simulink model "CSE1_Oculus_gesture"  (R2014a)
settings: Solver=ode4  StartTime=0.0  StopTime=inf  FixedStep=0.01  RelTol=1e-3
undefined symbols (not defined in the file): v_max
libraries: marine_gnc x11
(part 1 of 4)
settings Model: Creator=mclab  LastModifiedBy=mclab
settings RTWCC: SystemTargetFile=NIVeriStand_VxWorks.tlc  TemplateMakefile=NIVeriStand_VxWorks.tmf  Description=NI VeriStand VxWorks Real-Time Target for Release 2007b or later  ProcessScript=NIVeriStand_VxWorks_make_rtw_hook
settings STFCustomTargetCC: ConcurrentExecutionCompliant=off  MatFileLogging=on  MATLABClassNameForMDSCustomization=Simulink.SoftwareTarget.TargetSpecificTriggerConfigurationBase  SystemTargetFile=NIVeriStand_VxWorks.tlc

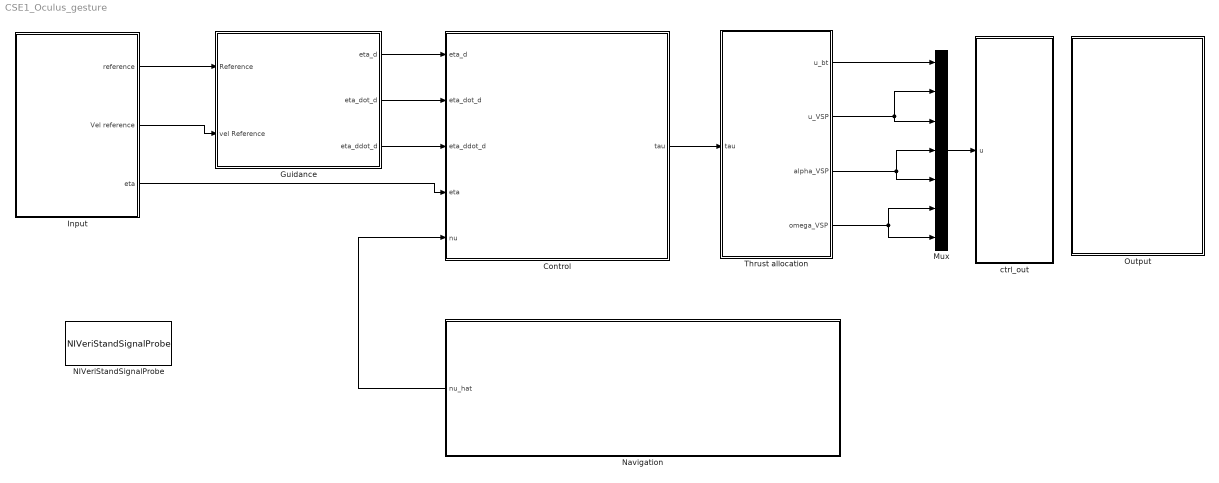
== system CSE1_Oculus_gesture ==
  Control : Subsystem
  Guidance : Subsystem
  Input : Subsystem
  Mux : Mux  Inputs=7
  NIVeriStandSignalProbe : S-Function  FunctionName=NIVeriStandSignalProbe  Parameters=1  EnableBusSupport=off
  "Navigation " : Subsystem
  Output : Subsystem
  Thrust allocation : Subsystem
  ctrl_out : Subsystem
  wires:
  Control/1(tau) -> Thrust allocation/1(tau)
  Input/1(reference) -> Guidance/1("Reference ")
  Guidance/1(eta_d) -> Control/1(eta_d)
  Guidance/3(eta_ddot_d) -> Control/3(eta_ddot_d)
  Guidance/2(eta_dot_d) -> Control/2(eta_dot_d)
  Input/3(eta) -> Control/4(eta)
  Thrust allocation/1(u_bt) -> Mux/1
  Thrust allocation/2(u_VSP) -> Mux/2, Mux/3
  Thrust allocation/3(alpha_VSP) -> Mux/4, Mux/5
  Thrust allocation/4(omega_VSP) -> Mux/6, Mux/7
  "Navigation "/1(nu_hat) -> Control/5(nu)
  Input/2(Vel reference) -> Guidance/2("vel Reference ")
  Mux/1 -> ctrl_out/1(u)

== system CSE1_Oculus_gesture/Control ==
  eta_d : Inport
  eta_dot_d : Inport  Port=2
  eta_ddot_d : Inport  Port=3
  eta : Inport  Port=4
  nu : Inport  Port=5
  DP Controller : Subsystem
  Terminator : Terminator
  tau : Outport
  tag scope: tau=global
  wires:
  eta_d/1 -> DP Controller/1(eta_d)
  eta/1 -> DP Controller/2(eta)
  nu/1 -> DP Controller/3(nu)
  DP Controller/1(tau) -> [tau], tau/1
  eta_ddot_d/1 -> Terminator/1
  eta_dot_d/1 -> DP Controller/4(eta_dot_d)

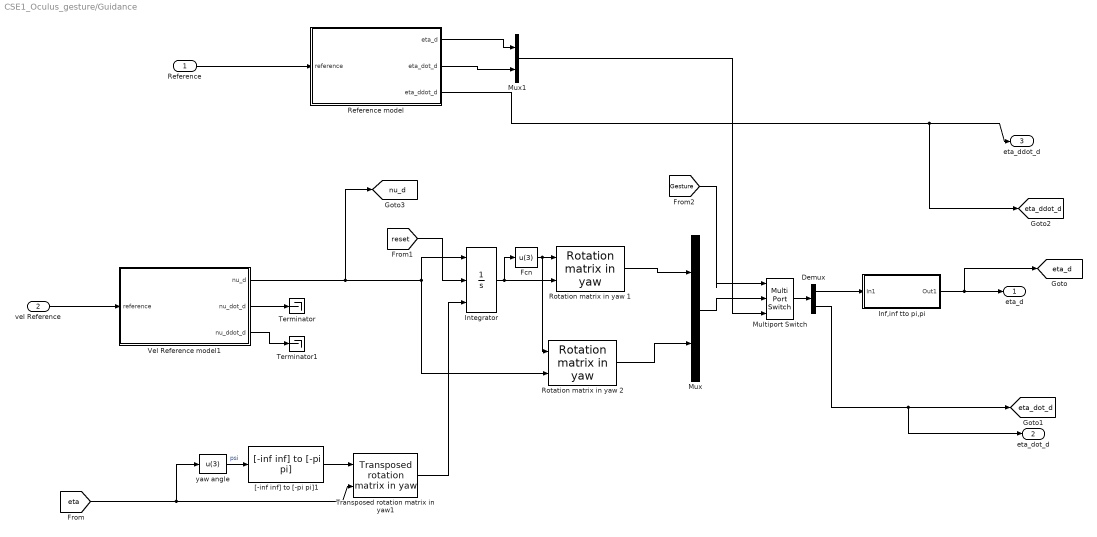
== system CSE1_Oculus_gesture/Guidance ==
  "Reference " : Inport
  "vel Reference " : Inport  Port=2
  Demux : Demux  Outputs=2
  Fcn : Fcn  Expr=u(3)
  Inf,inf tto pi,pi : Subsystem
  Integrator : Integrator  ExternalReset=either  InitialConditionSource=external
  Multiport Switch : MultiPortSwitch  DataPortOrder=Zero-based contiguous  Inputs=2
  Mux : Mux  Inputs=2
  Mux1 : Mux  Inputs=2
  Reference model : Subsystem
  Rotation matrix in yaw 1 : marine_gnc/Models/ Kinematics/Rotation matrix in yaw 
  Rotation matrix in yaw 2 : marine_gnc/Models/ Kinematics/Rotation matrix in yaw 
  Terminator : Terminator
  Terminator1 : Terminator
  Transposed rotation matrix in yaw1 : marine_gnc/Models/ Kinematics/Transposed rotation  matrix in yaw
  Vel Reference model1 : Subsystem
  "[-inf inf] to [-pi pi]1" : marine_gnc/Utilities/Math Operations/[-inf inf] to [-pi pi]
  yaw angle : Fcn  Expr=u(3)
  eta_d : Outport
  eta_dot_d : Outport  Port=2
  eta_ddot_d : Outport  Port=3
  tag scope: eta_d=global, eta_ddot_d=global, eta_dot_d=global, nu_d=global
  wires:
  Demux/1 -> Inf,inf tto pi,pi/1(In1)
  Demux/2 -> eta_dot_d/1, [eta_dot_d]
  Reference model/3(eta_ddot_d) -> [eta_ddot_d], eta_ddot_d/1
  "Reference "/1 -> Reference model/1(reference)
  "vel Reference "/1 -> Vel Reference model1/1(reference)
  Integrator/1 -> Fcn/1, Rotation matrix in yaw 1/2
  Rotation matrix in yaw 1/1 -> Mux/1
  Vel Reference model1/1(nu_d) -> Rotation matrix in yaw 2/2, Integrator/1, [nu_d]
  Fcn/1 -> Rotation matrix in yaw 2/1, Rotation matrix in yaw 1/1
  Rotation matrix in yaw 2/1 -> Mux/2
  Transposed rotation matrix in yaw1/1 -> Integrator/3
  [reset] -> Integrator/2
  "[-inf inf] to [-pi pi]1"/1 -> Transposed rotation matrix in yaw1/1
  yaw angle/1 -> "[-inf inf] to [-pi pi]1"/1  "psi"
  [eta] -> yaw angle/1, Transposed rotation matrix in yaw1/2
  Reference model/2(eta_dot_d) -> Mux1/2
  Reference model/1(eta_d) -> Mux1/1
  Multiport Switch/1 -> Demux/1
  Mux1/1 -> Multiport Switch/3
  Mux/1 -> Multiport Switch/2
  [Gesture] -> Multiport Switch/1
  Vel Reference model1/2(nu_dot_d) -> Terminator/1
  Vel Reference model1/3(nu_ddot_d) -> Terminator1/1
  Inf,inf tto pi,pi/1(Out1) -> [eta_d], eta_d/1

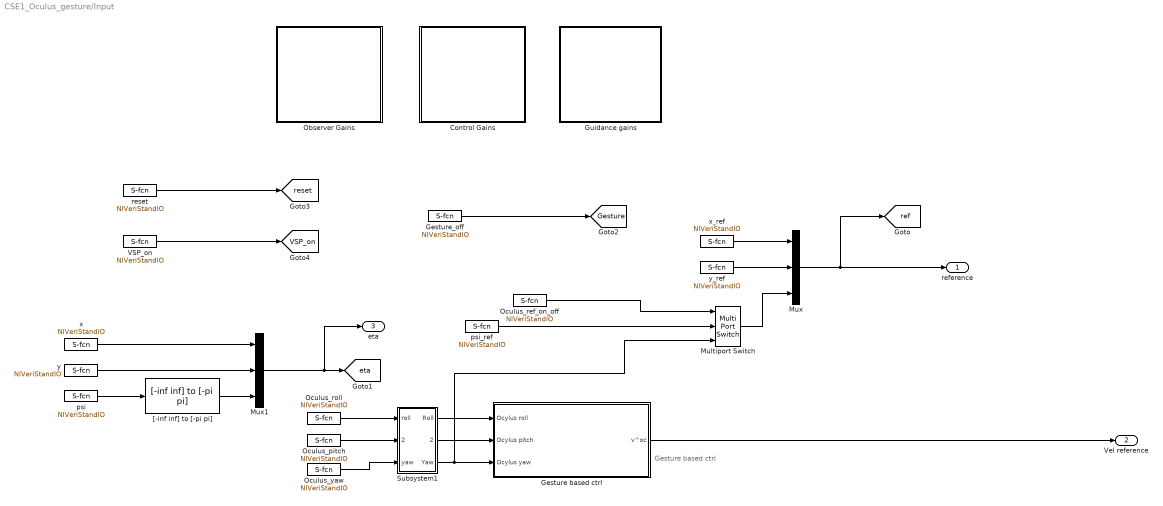
== system CSE1_Oculus_gesture/Input ==
  note: Gesture based ctrl
  Control Gains : Subsystem
  Gesture based ctrl : Subsystem
  Gesture_off : S-Function  Priority=11  FunctionName=NIVeriStandIO  Parameters=width dtype portnum stime stype btype  EnableBusSupport=off  mask(NI VeriStand Inport){portnum=11, width=-1, stime=-1, dtype=auto, stype=auto, btype=1}
      mask prompts: portnum "Port number:"; width "Port dimensions (-1 for dynamically sized):"; stime "Sample time (-1 for inherited):"; dtype "Data type:"; stype "Signal type:"; btype "Block type:"
      mask help: Use this inport on any level of nested subsystems to allow NI VeriStand software to map signals to it.
      mask init:
      | NIVeriStandIO_init;
      settings: CopyFcn=NIVeriStand_MDL_functions('', 'IO_copy');  DeleteFcn=NIVeriStand_MDL_functions('', 'IO_delete');  MoveFcn=set_param(gcb, 'Mask', 'on');
      mask Callback portnum: NIVeriStand_MDL_functions('', 'IO_setportnum');
      mask TypeOptions dtype: auto | double | single | int8 | uint8 | int16 | uint16 | int32 | uint32 | boolean
      mask Callback dtype: NIVeriStand_MDL_functions('', 'IO_booleansignal');
      mask TypeOptions stype: auto | real | complex
      mask Display:
      | patch([-x x], [-y y], [.90980 .81960 .32156]);
      | plot([xrad -x x xrad], [yrad -y y yrad]);
      | fprintf('NI In%d', portnum);
  Guidance gains : Subsystem
  Multiport Switch : MultiPortSwitch  DataPortOrder=Zero-based contiguous  Inputs=2
  Mux : Mux  Inputs=3
  Mux1 : Mux  Inputs=3
  Observer Gains : Subsystem
  Oculus_pitch : S-Function  Priority=12  FunctionName=NIVeriStandIO  Parameters=width dtype portnum stime stype btype  EnableBusSupport=off  mask(NI VeriStand Inport){portnum=12, width=-1, stime=-1, dtype=auto, stype=auto, btype=1}
      mask prompts: portnum "Port number:"; width "Port dimensions (-1 for dynamically sized):"; stime "Sample time (-1 for inherited):"; dtype "Data type:"; stype "Signal type:"; btype "Block type:"
      mask help: Use this inport on any level of nested subsystems to allow NI VeriStand software to map signals to it.
      mask init:
      | NIVeriStandIO_init;
      settings: CopyFcn=NIVeriStand_MDL_functions('', 'IO_copy');  DeleteFcn=NIVeriStand_MDL_functions('', 'IO_delete');  MoveFcn=set_param(gcb, 'Mask', 'on');
      mask Callback portnum: NIVeriStand_MDL_functions('', 'IO_setportnum');
      mask TypeOptions dtype: auto | double | single | int8 | uint8 | int16 | uint16 | int32 | uint32 | boolean
      mask Callback dtype: NIVeriStand_MDL_functions('', 'IO_booleansignal');
      mask TypeOptions stype: auto | real | complex
      mask Display:
      | patch([-x x], [-y y], [.90980 .81960 .32156]);
      | plot([xrad -x x xrad], [yrad -y y yrad]);
      | fprintf('NI In%d', portnum);
  Oculus_ref_on_off : S-Function  Priority=3  FunctionName=NIVeriStandIO  Parameters=width dtype portnum stime stype btype  EnableBusSupport=off  mask(NI VeriStand Inport){portnum=3, width=-1, stime=-1, dtype=auto, stype=auto, btype=1}
      mask prompts: portnum "Port number:"; width "Port dimensions (-1 for dynamically sized):"; stime "Sample time (-1 for inherited):"; dtype "Data type:"; stype "Signal type:"; btype "Block type:"
      mask help: Use this inport on any level of nested subsystems to allow NI VeriStand software to map signals to it.
      mask init:
      | NIVeriStandIO_init;
      settings: CopyFcn=NIVeriStand_MDL_functions('', 'IO_copy');  DeleteFcn=NIVeriStand_MDL_functions('', 'IO_delete');  MoveFcn=set_param(gcb, 'Mask', 'on');
      mask Callback portnum: NIVeriStand_MDL_functions('', 'IO_setportnum');
      mask TypeOptions dtype: auto | double | single | int8 | uint8 | int16 | uint16 | int32 | uint32 | boolean
      mask Callback dtype: NIVeriStand_MDL_functions('', 'IO_booleansignal');
      mask TypeOptions stype: auto | real | complex
      mask Display:
      | patch([-x x], [-y y], [.90980 .81960 .32156]);
      | plot([xrad -x x xrad], [yrad -y y yrad]);
      | fprintf('NI In%d', portnum);
  Oculus_roll : S-Function  Priority=13  FunctionName=NIVeriStandIO  Parameters=width dtype portnum stime stype btype  EnableBusSupport=off  mask(NI VeriStand Inport){portnum=13, width=-1, stime=-1, dtype=auto, stype=auto, btype=1}
      mask prompts: portnum "Port number:"; width "Port dimensions (-1 for dynamically sized):"; stime "Sample time (-1 for inherited):"; dtype "Data type:"; stype "Signal type:"; btype "Block type:"
      mask help: Use this inport on any level of nested subsystems to allow NI VeriStand software to map signals to it.
      mask init:
      | NIVeriStandIO_init;
      settings: CopyFcn=NIVeriStand_MDL_functions('', 'IO_copy');  DeleteFcn=NIVeriStand_MDL_functions('', 'IO_delete');  MoveFcn=set_param(gcb, 'Mask', 'on');
      mask Callback portnum: NIVeriStand_MDL_functions('', 'IO_setportnum');
      mask TypeOptions dtype: auto | double | single | int8 | uint8 | int16 | uint16 | int32 | uint32 | boolean
      mask Callback dtype: NIVeriStand_MDL_functions('', 'IO_booleansignal');
      mask TypeOptions stype: auto | real | complex
      mask Display:
      | patch([-x x], [-y y], [.90980 .81960 .32156]);
      | plot([xrad -x x xrad], [yrad -y y yrad]);
      | fprintf('NI In%d', portnum);
  Oculus_yaw : S-Function  Priority=5  FunctionName=NIVeriStandIO  Parameters=width dtype portnum stime stype btype  EnableBusSupport=off  mask(NI VeriStand Inport){portnum=5, width=-1, stime=-1, dtype=auto, stype=auto, btype=1}
      mask prompts: portnum "Port number:"; width "Port dimensions (-1 for dynamically sized):"; stime "Sample time (-1 for inherited):"; dtype "Data type:"; stype "Signal type:"; btype "Block type:"
      mask help: Use this inport on any level of nested subsystems to allow NI VeriStand software to map signals to it.
      mask init:
      | NIVeriStandIO_init;
      settings: CopyFcn=NIVeriStand_MDL_functions('', 'IO_copy');  DeleteFcn=NIVeriStand_MDL_functions('', 'IO_delete');  MoveFcn=set_param(gcb, 'Mask', 'on');
      mask Callback portnum: NIVeriStand_MDL_functions('', 'IO_setportnum');
      mask TypeOptions dtype: auto | double | single | int8 | uint8 | int16 | uint16 | int32 | uint32 | boolean
      mask Callback dtype: NIVeriStand_MDL_functions('', 'IO_booleansignal');
      mask TypeOptions stype: auto | real | complex
      mask Display:
      | patch([-x x], [-y y], [.90980 .81960 .32156]);
      | plot([xrad -x x xrad], [yrad -y y yrad]);
      | fprintf('NI In%d', portnum);
  Subsystem1 : Subsystem
  VSP_on : S-Function  Priority=2  FunctionName=NIVeriStandIO  Parameters=width dtype portnum stime stype btype  EnableBusSupport=off  mask(NI VeriStand Inport){portnum=2, width=-1, stime=-1, dtype=auto, stype=auto, btype=1}
      mask prompts: portnum "Port number:"; width "Port dimensions (-1 for dynamically sized):"; stime "Sample time (-1 for inherited):"; dtype "Data type:"; stype "Signal type:"; btype "Block type:"
      mask help: Use this inport on any level of nested subsystems to allow NI VeriStand software to map signals to it.
      mask init:
      | NIVeriStandIO_init;
      settings: CopyFcn=NIVeriStand_MDL_functions('', 'IO_copy');  DeleteFcn=NIVeriStand_MDL_functions('', 'IO_delete');  MoveFcn=set_param(gcb, 'Mask', 'on');
      mask Callback portnum: NIVeriStand_MDL_functions('', 'IO_setportnum');
      mask TypeOptions dtype: auto | double | single | int8 | uint8 | int16 | uint16 | int32 | uint32 | boolean
      mask Callback dtype: NIVeriStand_MDL_functions('', 'IO_booleansignal');
      mask TypeOptions stype: auto | real | complex
      mask Display:
      | patch([-x x], [-y y], [.90980 .81960 .32156]);
      | plot([xrad -x x xrad], [yrad -y y yrad]);
      | fprintf('NI In%d', portnum);
  "[-inf inf] to [-pi pi]" : marine_gnc/Utilities/Math Operations/[-inf inf] to [-pi pi]
  psi : S-Function  Priority=10  FunctionName=NIVeriStandIO  Parameters=width dtype portnum stime stype btype  EnableBusSupport=off  mask(NI VeriStand Inport){portnum=10, width=-1, stime=-1, dtype=auto, stype=auto, btype=1}
      mask prompts: portnum "Port number:"; width "Port dimensions (-1 for dynamically sized):"; stime "Sample time (-1 for inherited):"; dtype "Data type:"; stype "Signal type:"; btype "Block type:"
      mask help: Use this inport on any level of nested subsystems to allow NI VeriStand software to map signals to it.
      mask init:
      | NIVeriStandIO_init;
      settings: CopyFcn=NIVeriStand_MDL_functions('', 'IO_copy');  DeleteFcn=NIVeriStand_MDL_functions('', 'IO_delete');  MoveFcn=set_param(gcb, 'Mask', 'on');
      mask Callback portnum: NIVeriStand_MDL_functions('', 'IO_setportnum');
      mask TypeOptions dtype: auto | double | single | int8 | uint8 | int16 | uint16 | int32 | uint32 | boolean
      mask Callback dtype: NIVeriStand_MDL_functions('', 'IO_booleansignal');
      mask TypeOptions stype: auto | real | complex
      mask Display:
      | patch([-x x], [-y y], [.90980 .81960 .32156]);
      | plot([xrad -x x xrad], [yrad -y y yrad]);
      | fprintf('NI In%d', portnum);
  psi_ref : S-Function  Priority=4  FunctionName=NIVeriStandIO  Parameters=width dtype portnum stime stype btype  EnableBusSupport=off  mask(NI VeriStand Inport){portnum=4, width=-1, stime=-1, dtype=auto, stype=auto, btype=1}
      mask prompts: portnum "Port number:"; width "Port dimensions (-1 for dynamically sized):"; stime "Sample time (-1 for inherited):"; dtype "Data type:"; stype "Signal type:"; btype "Block type:"
      mask help: Use this inport on any level of nested subsystems to allow NI VeriStand software to map signals to it.
      mask init:
      | NIVeriStandIO_init;
      settings: CopyFcn=NIVeriStand_MDL_functions('', 'IO_copy');  DeleteFcn=NIVeriStand_MDL_functions('', 'IO_delete');  MoveFcn=set_param(gcb, 'Mask', 'on');
      mask Callback portnum: NIVeriStand_MDL_functions('', 'IO_setportnum');
      mask TypeOptions dtype: auto | double | single | int8 | uint8 | int16 | uint16 | int32 | uint32 | boolean
      mask Callback dtype: NIVeriStand_MDL_functions('', 'IO_booleansignal');
      mask TypeOptions stype: auto | real | complex
      mask Display:
      | patch([-x x], [-y y], [.90980 .81960 .32156]);
      | plot([xrad -x x xrad], [yrad -y y yrad]);
      | fprintf('NI In%d', portnum);
  reset : S-Function  Priority=1  FunctionName=NIVeriStandIO  Parameters=width dtype portnum stime stype btype  EnableBusSupport=off  mask(NI VeriStand Inport){portnum=1, width=-1, stime=-1, dtype=auto, stype=auto, btype=1}
      mask prompts: portnum "Port number:"; width "Port dimensions (-1 for dynamically sized):"; stime "Sample time (-1 for inherited):"; dtype "Data type:"; stype "Signal type:"; btype "Block type:"
      mask help: Use this inport on any level of nested subsystems to allow NI VeriStand software to map signals to it.
      mask init:
      | NIVeriStandIO_init;
      settings: CopyFcn=NIVeriStand_MDL_functions('', 'IO_copy');  DeleteFcn=NIVeriStand_MDL_functions('', 'IO_delete');  MoveFcn=set_param(gcb, 'Mask', 'on');
      mask Callback portnum: NIVeriStand_MDL_functions('', 'IO_setportnum');
      mask TypeOptions dtype: auto | double | single | int8 | uint8 | int16 | uint16 | int32 | uint32 | boolean
      mask Callback dtype: NIVeriStand_MDL_functions('', 'IO_booleansignal');
      mask TypeOptions stype: auto | real | complex
      mask Display:
      | patch([-x x], [-y y], [.90980 .81960 .32156]);
      | plot([xrad -x x xrad], [yrad -y y yrad]);
      | fprintf('NI In%d', portnum);
  x : S-Function  Priority=8  FunctionName=NIVeriStandIO  Parameters=width dtype portnum stime stype btype  EnableBusSupport=off  mask(NI VeriStand Inport){portnum=8, width=-1, stime=-1, dtype=auto, stype=auto, btype=1}
      mask prompts: portnum "Port number:"; width "Port dimensions (-1 for dynamically sized):"; stime "Sample time (-1 for inherited):"; dtype "Data type:"; stype "Signal type:"; btype "Block type:"
      mask help: Use this inport on any level of nested subsystems to allow NI VeriStand software to map signals to it.
      mask init:
      | NIVeriStandIO_init;
      settings: CopyFcn=NIVeriStand_MDL_functions('', 'IO_copy');  DeleteFcn=NIVeriStand_MDL_functions('', 'IO_delete');  MoveFcn=set_param(gcb, 'Mask', 'on');
      mask Callback portnum: NIVeriStand_MDL_functions('', 'IO_setportnum');
      mask TypeOptions dtype: auto | double | single | int8 | uint8 | int16 | uint16 | int32 | uint32 | boolean
      mask Callback dtype: NIVeriStand_MDL_functions('', 'IO_booleansignal');
      mask TypeOptions stype: auto | real | complex
      mask Display:
      | patch([-x x], [-y y], [.90980 .81960 .32156]);
      | plot([xrad -x x xrad], [yrad -y y yrad]);
      | fprintf('NI In%d', portnum);
  x_ref : S-Function  Priority=6  FunctionName=NIVeriStandIO  Parameters=width dtype portnum stime stype btype  EnableBusSupport=off  mask(NI VeriStand Inport){portnum=6, width=-1, stime=-1, dtype=auto, stype=auto, btype=1}
      mask prompts: portnum "Port number:"; width "Port dimensions (-1 for dynamically sized):"; stime "Sample time (-1 for inherited):"; dtype "Data type:"; stype "Signal type:"; btype "Block type:"
      mask help: Use this inport on any level of nested subsystems to allow NI VeriStand software to map signals to it.
      mask init:
      | NIVeriStandIO_init;
      settings: CopyFcn=NIVeriStand_MDL_functions('', 'IO_copy');  DeleteFcn=NIVeriStand_MDL_functions('', 'IO_delete');  MoveFcn=set_param(gcb, 'Mask', 'on');
      mask Callback portnum: NIVeriStand_MDL_functions('', 'IO_setportnum');
      mask TypeOptions dtype: auto | double | single | int8 | uint8 | int16 | uint16 | int32 | uint32 | boolean
      mask Callback dtype: NIVeriStand_MDL_functions('', 'IO_booleansignal');
      mask TypeOptions stype: auto | real | complex
      mask Display:
      | patch([-x x], [-y y], [.90980 .81960 .32156]);
      | plot([xrad -x x xrad], [yrad -y y yrad]);
      | fprintf('NI In%d', portnum);
  y : S-Function  Priority=9  FunctionName=NIVeriStandIO  Parameters=width dtype portnum stime stype btype  EnableBusSupport=off  mask(NI VeriStand Inport){portnum=9, width=-1, stime=-1, dtype=auto, stype=auto, btype=1}
      mask prompts: portnum "Port number:"; width "Port dimensions (-1 for dynamically sized):"; stime "Sample time (-1 for inherited):"; dtype "Data type:"; stype "Signal type:"; btype "Block type:"
      mask help: Use this inport on any level of nested subsystems to allow NI VeriStand software to map signals to it.
      mask init:
      | NIVeriStandIO_init;
      settings: CopyFcn=NIVeriStand_MDL_functions('', 'IO_copy');  DeleteFcn=NIVeriStand_MDL_functions('', 'IO_delete');  MoveFcn=set_param(gcb, 'Mask', 'on');
      mask Callback portnum: NIVeriStand_MDL_functions('', 'IO_setportnum');
      mask TypeOptions dtype: auto | double | single | int8 | uint8 | int16 | uint16 | int32 | uint32 | boolean
      mask Callback dtype: NIVeriStand_MDL_functions('', 'IO_booleansignal');
      mask TypeOptions stype: auto | real | complex
      mask Display:
      | patch([-x x], [-y y], [.90980 .81960 .32156]);
      | plot([xrad -x x xrad], [yrad -y y yrad]);
      | fprintf('NI In%d', portnum);
  y_ref : S-Function  Priority=7  FunctionName=NIVeriStandIO  Parameters=width dtype portnum stime stype btype  EnableBusSupport=off  mask(NI VeriStand Inport){portnum=7, width=-1, stime=-1, dtype=auto, stype=auto, btype=1}
      mask prompts: portnum "Port number:"; width "Port dimensions (-1 for dynamically sized):"; stime "Sample time (-1 for inherited):"; dtype "Data type:"; stype "Signal type:"; btype "Block type:"
      mask help: Use this inport on any level of nested subsystems to allow NI VeriStand software to map signals to it.
      mask init:
      | NIVeriStandIO_init;
      settings: CopyFcn=NIVeriStand_MDL_functions('', 'IO_copy');  DeleteFcn=NIVeriStand_MDL_functions('', 'IO_delete');  MoveFcn=set_param(gcb, 'Mask', 'on');
      mask Callback portnum: NIVeriStand_MDL_functions('', 'IO_setportnum');
      mask TypeOptions dtype: auto | double | single | int8 | uint8 | int16 | uint16 | int32 | uint32 | boolean
      mask Callback dtype: NIVeriStand_MDL_functions('', 'IO_booleansignal');
      mask TypeOptions stype: auto | real | complex
      mask Display:
      | patch([-x x], [-y y], [.90980 .81960 .32156]);
      | plot([xrad -x x xrad], [yrad -y y yrad]);
      | fprintf('NI In%d', portnum);
  reference : Outport
  Vel reference : Outport  Port=2
  eta : Outport  Port=3
  tag scope: Gesture=global, VSP_on=global, eta=global, ref=global, reset=global
  wires:
  Mux/1 -> [ref], reference/1
  reset/1 -> [reset]
  VSP_on/1 -> [VSP_on]
  x_ref/1 -> Mux/1
  y_ref/1 -> Mux/2
  psi_ref/1 -> Multiport Switch/2
  psi/1 -> "[-inf inf] to [-pi pi]"/1
  Mux1/1 -> eta/1, [eta]
  Multiport Switch/1 -> Mux/3
  Oculus_ref_on_off/1 -> Multiport Switch/1
  y/1 -> Mux1/2
  x/1 -> Mux1/1
  Gesture based ctrl/1("v^oc ") -> Vel reference/1
  Gesture_off/1 -> [Gesture]
  "[-inf inf] to [-pi pi]"/1 -> Mux1/3
  Subsystem1/3(Yaw) -> Multiport Switch/3, Gesture based ctrl/3(Ocylus yaw)
  Oculus_roll/1 -> Subsystem1/1(roll)
  Oculus_pitch/1 -> Subsystem1/2(pitch)
  Oculus_yaw/1 -> Subsystem1/3(yaw)
  Subsystem1/1(Roll) -> Gesture based ctrl/1(Ocylus roll)
  Subsystem1/2(Pitch) -> Gesture based ctrl/2(Ocylus pitch)

== system CSE1_Oculus_gesture/Navigation  ==
  Derivative filter : Subsystem
  nu_hat : Outport
  tag scope: nu_hat=global
  wires:
  [eta] -> Derivative filter/1(eta)
  Derivative filter/1(nu_hat) -> nu_hat/1, [nu_hat]

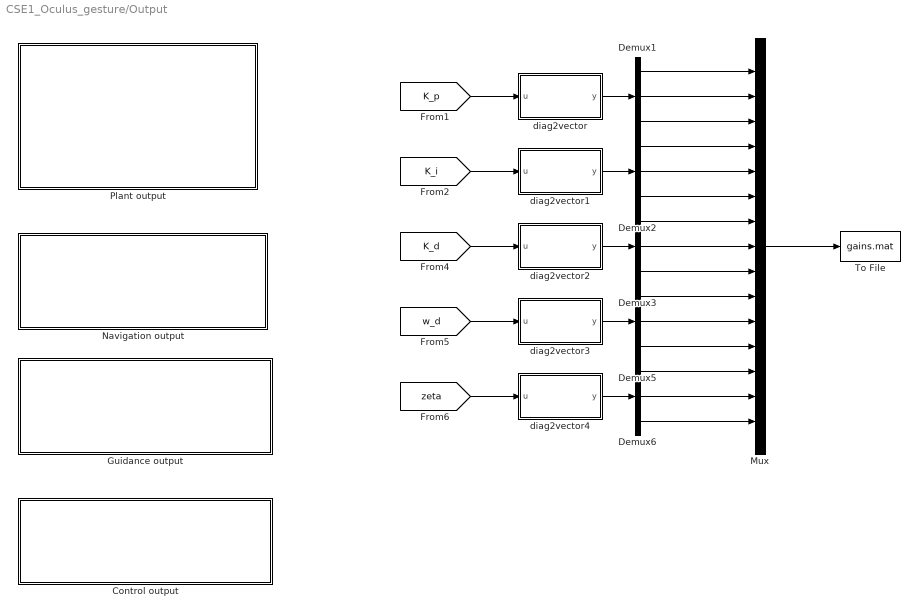
== system CSE1_Oculus_gesture/Output ==
  Control output : Subsystem
  Demux{1..3,5..6} (5 alike) : Demux  Outputs=3
  Guidance output : Subsystem
  Mux : Mux  Inputs=15
  Navigation output : Subsystem
  Plant output : Subsystem
  To File : ToFile  Filename=gains.mat
  diag2vector : MATLAB Function  TreatAsAtomicUnit=on
  diag2vector1 : MATLAB Function  TreatAsAtomicUnit=on
  diag2vector2 : MATLAB Function  TreatAsAtomicUnit=on
  diag2vector3 : MATLAB Function  TreatAsAtomicUnit=on
  diag2vector4 : MATLAB Function  TreatAsAtomicUnit=on
  wires:
  Mux/1 -> To File/1
  [K_p] -> diag2vector/1(u)
  diag2vector/1(y) -> Demux1/1
  Demux1/1 -> Mux/1
  Demux1/2 -> Mux/2
  Demux1/3 -> Mux/3
  [K_i] -> diag2vector1/1(u)
  diag2vector1/1(y) -> Demux2/1
  Demux2/1 -> Mux/4
  Demux2/2 -> Mux/5
  Demux2/3 -> Mux/6
  [K_d] -> diag2vector2/1(u)
  diag2vector2/1(y) -> Demux3/1
  Demux3/1 -> Mux/7
  Demux3/2 -> Mux/8
  Demux3/3 -> Mux/9
  [w_d] -> diag2vector3/1(u)
  diag2vector3/1(y) -> Demux5/1
  Demux5/1 -> Mux/10
  Demux5/2 -> Mux/11
  Demux5/3 -> Mux/12
  [zeta] -> diag2vector4/1(u)
  diag2vector4/1(y) -> Demux6/1
  Demux6/1 -> Mux/13
  Demux6/2 -> Mux/14
  Demux6/3 -> Mux/15

== system CSE1_Oculus_gesture/Thrust allocation ==
  tau : Inport
  Demux : Demux  Outputs=3
  Mux1 : Mux  Inputs=3
  Thrust allocation : MATLAB Function  TreatAsAtomicUnit=on
  u_bt : Outport
  u_VSP : Outport  Port=2
  alpha_VSP : Outport  Port=3
  omega_VSP : Outport  Port=4
  tag scope: thrust=global
  wires:
  [VSP_on] -> Thrust allocation/4(VSP_on)
  Demux/1 -> Thrust allocation/1(X)
  Demux/3 -> Thrust allocation/3(N)
  Thrust allocation/4(omega_VSP) -> omega_VSP/1
  Demux/2 -> Thrust allocation/2(Y)
  tau/1 -> Demux/1
  Thrust allocation/1(u_BT) -> u_bt/1, Mux1/1
  Thrust allocation/2(u_VSP) -> u_VSP/1, Mux1/2
  Thrust allocation/3(alpha_VSP) -> alpha_VSP/1, Mux1/3
  Mux1/1 -> [thrust]

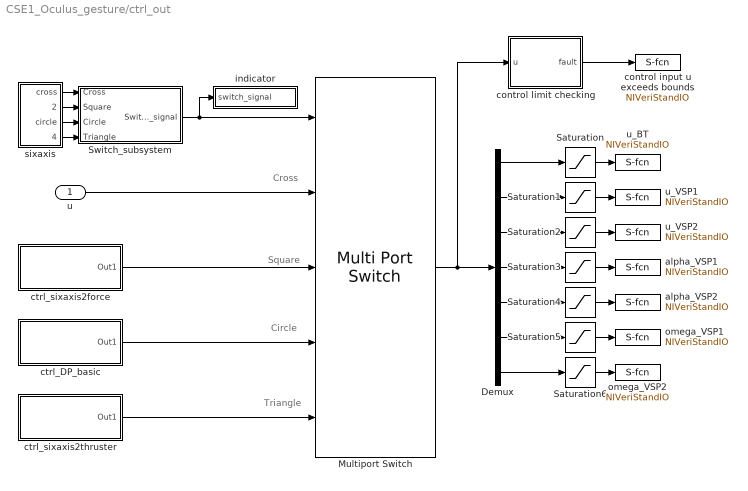
== system CSE1_Oculus_gesture/ctrl_out ==
  note: Cross
  note: Square
  note: Circle
  note: Triangle
  u : Inport
  Demux : Demux  Outputs=7
  Multiport Switch : MultiPortSwitch  Inputs=4
  Saturation : Saturate  UpperLimit=1  LowerLimit=-1
  Saturation1 : Saturate  UpperLimit=1  LowerLimit=0
  Saturation2 : Saturate  UpperLimit=1  LowerLimit=0
  Saturation3 : Saturate  UpperLimit=pi  LowerLimit=-pi
  Saturation4 : Saturate  UpperLimit=pi  LowerLimit=-pi
  Saturation5 : Saturate  UpperLimit=1  LowerLimit=-1
  Saturation6 : Saturate  UpperLimit=1  LowerLimit=-1
  Switch_subsystem : Subsystem
  alpha_VSP1 : S-Function  Priority=5  FunctionName=NIVeriStandIO  Parameters=width dtype portnum stime stype btype  EnableBusSupport=off  mask(NI VeriStand Outport){portnum=5, width=-1, stime=-1, dtype=auto, stype=auto, btype=0}
      mask prompts: portnum "Port number:"; width "Port dimensions (-1 for dynamically sized):"; stime "Sample time (-1 for inherited):"; dtype "Data type:"; stype "Signal type:"; btype "Block type:"
      mask help: Use this outport on any level of nested subsystems to allow NI VeriStand software to map signals to it.
      mask init:
      | NIVeriStandIO_init;
      settings: CopyFcn=NIVeriStand_MDL_functions('', 'IO_copy');  DeleteFcn=NIVeriStand_MDL_functions('', 'IO_delete');  MoveFcn=set_param(gcb, 'Mask', 'on');
      mask Callback portnum: NIVeriStand_MDL_functions('', 'IO_setportnum');
      mask TypeOptions dtype: auto | double | single | int8 | uint8 | int16 | uint16 | int32 | uint32 | boolean
      mask Callback dtype: NIVeriStand_MDL_functions('', 'IO_booleansignal');
      mask TypeOptions stype: auto | real | complex
      mask Display:
      | patch([-x x], [-y y], [.90980 .81960 .32156]);
      | plot([xrad -x x xrad], [yrad -y y yrad]);
      | fprintf('NI Out%d', portnum);
  alpha_VSP2 : S-Function  Priority=1  FunctionName=NIVeriStandIO  Parameters=width dtype portnum stime stype btype  EnableBusSupport=off  mask(NI VeriStand Outport){portnum=1, width=-1, stime=-1, dtype=auto, stype=auto, btype=0}
      mask prompts: portnum "Port number:"; width "Port dimensions (-1 for dynamically sized):"; stime "Sample time (-1 for inherited):"; dtype "Data type:"; stype "Signal type:"; btype "Block type:"
      mask help: Use this outport on any level of nested subsystems to allow NI VeriStand software to map signals to it.
      mask init:
      | NIVeriStandIO_init;
      settings: CopyFcn=NIVeriStand_MDL_functions('', 'IO_copy');  DeleteFcn=NIVeriStand_MDL_functions('', 'IO_delete');  MoveFcn=set_param(gcb, 'Mask', 'on');
      mask Callback portnum: NIVeriStand_MDL_functions('', 'IO_setportnum');
      mask TypeOptions dtype: auto | double | single | int8 | uint8 | int16 | uint16 | int32 | uint32 | boolean
      mask Callback dtype: NIVeriStand_MDL_functions('', 'IO_booleansignal');
      mask TypeOptions stype: auto | real | complex
      mask Display:
      | patch([-x x], [-y y], [.90980 .81960 .32156]);
      | plot([xrad -x x xrad], [yrad -y y yrad]);
      | fprintf('NI Out%d', portnum);
  control input u exceeds bounds : S-Function  Priority=8  FunctionName=NIVeriStandIO  Parameters=width dtype portnum stime stype btype  EnableBusSupport=off  mask(NI VeriStand Outport){portnum=8, width=-1, stime=-1, dtype=auto, stype=auto, btype=0}
      mask prompts: portnum "Port number:"; width "Port dimensions (-1 for dynamically sized):"; stime "Sample time (-1 for inherited):"; dtype "Data type:"; stype "Signal type:"; btype "Block type:"
      mask help: Use this outport on any level of nested subsystems to allow NI VeriStand software to map signals to it.
      mask init:
      | NIVeriStandIO_init;
      settings: CopyFcn=NIVeriStand_MDL_functions('', 'IO_copy');  DeleteFcn=NIVeriStand_MDL_functions('', 'IO_delete');  MoveFcn=set_param(gcb, 'Mask', 'on');
      mask Callback portnum: NIVeriStand_MDL_functions('', 'IO_setportnum');
      mask TypeOptions dtype: auto | double | single | int8 | uint8 | int16 | uint16 | int32 | uint32 | boolean
      mask Callback dtype: NIVeriStand_MDL_functions('', 'IO_booleansignal');
      mask TypeOptions stype: auto | real | complex
      mask Display:
      | patch([-x x], [-y y], [.90980 .81960 .32156]);
      | plot([xrad -x x xrad], [yrad -y y yrad]);
      | fprintf('NI Out%d', portnum);
  control limit checking : MATLAB Function  TreatAsAtomicUnit=on
  ctrl_DP_basic : Subsystem
  ctrl_sixaxis2force : Subsystem
  ctrl_sixaxis2thruster : Subsystem
  indicator : Subsystem
  omega_VSP1 : S-Function  Priority=6  FunctionName=NIVeriStandIO  Parameters=width dtype portnum stime stype btype  EnableBusSupport=off  mask(NI VeriStand Outport){portnum=6, width=-1, stime=-1, dtype=auto, stype=auto, btype=0}
      mask prompts: portnum "Port number:"; width "Port dimensions (-1 for dynamically sized):"; stime "Sample time (-1 for inherited):"; dtype "Data type:"; stype "Signal type:"; btype "Block type:"
      mask help: Use this outport on any level of nested subsystems to allow NI VeriStand software to map signals to it.
      mask init:
      | NIVeriStandIO_init;
      settings: CopyFcn=NIVeriStand_MDL_functions('', 'IO_copy');  DeleteFcn=NIVeriStand_MDL_functions('', 'IO_delete');  MoveFcn=set_param(gcb, 'Mask', 'on');
      mask Callback portnum: NIVeriStand_MDL_functions('', 'IO_setportnum');
      mask TypeOptions dtype: auto | double | single | int8 | uint8 | int16 | uint16 | int32 | uint32 | boolean
      mask Callback dtype: NIVeriStand_MDL_functions('', 'IO_booleansignal');
      mask TypeOptions stype: auto | real | complex
      mask Display:
      | patch([-x x], [-y y], [.90980 .81960 .32156]);
      | plot([xrad -x x xrad], [yrad -y y yrad]);
      | fprintf('NI Out%d', portnum);
  omega_VSP2 : S-Function  Priority=7  FunctionName=NIVeriStandIO  Parameters=width dtype portnum stime stype btype  EnableBusSupport=off  mask(NI VeriStand Outport){portnum=7, width=-1, stime=-1, dtype=auto, stype=auto, btype=0}
      mask prompts: portnum "Port number:"; width "Port dimensions (-1 for dynamically sized):"; stime "Sample time (-1 for inherited):"; dtype "Data type:"; stype "Signal type:"; btype "Block type:"
      mask help: Use this outport on any level of nested subsystems to allow NI VeriStand software to map signals to it.
      mask init:
      | NIVeriStandIO_init;
      settings: CopyFcn=NIVeriStand_MDL_functions('', 'IO_copy');  DeleteFcn=NIVeriStand_MDL_functions('', 'IO_delete');  MoveFcn=set_param(gcb, 'Mask', 'on');
      mask Callback portnum: NIVeriStand_MDL_functions('', 'IO_setportnum');
      mask TypeOptions dtype: auto | double | single | int8 | uint8 | int16 | uint16 | int32 | uint32 | boolean
      mask Callback dtype: NIVeriStand_MDL_functions('', 'IO_booleansignal');
      mask TypeOptions stype: auto | real | complex
      mask Display:
      | patch([-x x], [-y y], [.90980 .81960 .32156]);
      | plot([xrad -x x xrad], [yrad -y y yrad]);
      | fprintf('NI Out%d', portnum);
  sixaxis : Subsystem
  u_BT : S-Function  Priority=2  FunctionName=NIVeriStandIO  Parameters=width dtype portnum stime stype btype  EnableBusSupport=off  mask(NI VeriStand Outport){portnum=2, width=-1, stime=-1, dtype=auto, stype=auto, btype=0}
      mask prompts: portnum "Port number:"; width "Port dimensions (-1 for dynamically sized):"; stime "Sample time (-1 for inherited):"; dtype "Data type:"; stype "Signal type:"; btype "Block type:"
      mask help: Use this outport on any level of nested subsystems to allow NI VeriStand software to map signals to it.
      mask init:
      | NIVeriStandIO_init;
      settings: CopyFcn=NIVeriStand_MDL_functions('', 'IO_copy');  DeleteFcn=NIVeriStand_MDL_functions('', 'IO_delete');  MoveFcn=set_param(gcb, 'Mask', 'on');
      mask Callback portnum: NIVeriStand_MDL_functions('', 'IO_setportnum');
      mask TypeOptions dtype: auto | double | single | int8 | uint8 | int16 | uint16 | int32 | uint32 | boolean
      mask Callback dtype: NIVeriStand_MDL_functions('', 'IO_booleansignal');
      mask TypeOptions stype: auto | real | complex
      mask Display:
      | patch([-x x], [-y y], [.90980 .81960 .32156]);
      | plot([xrad -x x xrad], [yrad -y y yrad]);
      | fprintf('NI Out%d', portnum);
  u_VSP1 : S-Function  Priority=3  FunctionName=NIVeriStandIO  Parameters=width dtype portnum stime stype btype  EnableBusSupport=off  mask(NI VeriStand Outport){portnum=3, width=-1, stime=-1, dtype=auto, stype=auto, btype=0}
      mask prompts: portnum "Port number:"; width "Port dimensions (-1 for dynamically sized):"; stime "Sample time (-1 for inherited):"; dtype "Data type:"; stype "Signal type:"; btype "Block type:"
      mask help: Use this outport on any level of nested subsystems to allow NI VeriStand software to map signals to it.
      mask init:
      | NIVeriStandIO_init;
      settings: CopyFcn=NIVeriStand_MDL_functions('', 'IO_copy');  DeleteFcn=NIVeriStand_MDL_functions('', 'IO_delete');  MoveFcn=set_param(gcb, 'Mask', 'on');
      mask Callback portnum: NIVeriStand_MDL_functions('', 'IO_setportnum');
      mask TypeOptions dtype: auto | double | single | int8 | uint8 | int16 | uint16 | int32 | uint32 | boolean
      mask Callback dtype: NIVeriStand_MDL_functions('', 'IO_booleansignal');
      mask TypeOptions stype: auto | real | complex
      mask Display:
      | patch([-x x], [-y y], [.90980 .81960 .32156]);
      | plot([xrad -x x xrad], [yrad -y y yrad]);
      | fprintf('NI Out%d', portnum);
  u_VSP2 : S-Function  Priority=4  FunctionName=NIVeriStandIO  Parameters=width dtype portnum stime stype btype  EnableBusSupport=off  mask(NI VeriStand Outport){portnum=4, width=-1, stime=-1, dtype=auto, stype=auto, btype=0}
      mask prompts: portnum "Port number:"; width "Port dimensions (-1 for dynamically sized):"; stime "Sample time (-1 for inherited):"; dtype "Data type:"; stype "Signal type:"; btype "Block type:"
      mask help: Use this outport on any level of nested subsystems to allow NI VeriStand software to map signals to it.
      mask init:
      | NIVeriStandIO_init;
      settings: CopyFcn=NIVeriStand_MDL_functions('', 'IO_copy');  DeleteFcn=NIVeriStand_MDL_functions('', 'IO_delete');  MoveFcn=set_param(gcb, 'Mask', 'on');
      mask Callback portnum: NIVeriStand_MDL_functions('', 'IO_setportnum');
      mask TypeOptions dtype: auto | double | single | int8 | uint8 | int16 | uint16 | int32 | uint32 | boolean
      mask Callback dtype: NIVeriStand_MDL_functions('', 'IO_booleansignal');
      mask TypeOptions stype: auto | real | complex
      mask Display:
      | patch([-x x], [-y y], [.90980 .81960 .32156]);
      | plot([xrad -x x xrad], [yrad -y y yrad]);
      | fprintf('NI Out%d', portnum);
  wires:
  Multiport Switch/1 -> control limit checking/1(u), Demux/1
  Demux/1 -> Saturation/1
  Demux/2 -> Saturation1/1
  Demux/3 -> Saturation2/1
  Demux/4 -> Saturation3/1
  Demux/5 -> Saturation4/1
  Demux/6 -> Saturation5/1
  Demux/7 -> Saturation6/1
  Switch_subsystem/1(Switch_signal) -> indicator/1(switch_signal), Multiport Switch/1
  ctrl_sixaxis2thruster/1(Out1) -> Multiport Switch/5
  ctrl_DP_basic/1(Out1) -> Multiport Switch/4
  ctrl_sixaxis2force/1(Out1) -> Multiport Switch/3
  sixaxis/1(cross) -> Switch_subsystem/1(Cross)
  sixaxis/2(square) -> Switch_subsystem/2(Square)
  sixaxis/3(circle) -> Switch_subsystem/3(Circle)
  sixaxis/4(triangle) -> Switch_subsystem/4(Triangle)
  Saturation/1 -> u_BT/1
  Saturation1/1 -> u_VSP1/1
  Saturation2/1 -> u_VSP2/1
  Saturation3/1 -> alpha_VSP1/1
  Saturation4/1 -> alpha_VSP2/1
  Saturation5/1 -> omega_VSP1/1
  Saturation6/1 -> omega_VSP2/1
  control limit checking/1(fault) -> control input u exceeds bounds/1
  u/1 -> Multiport Switch/2

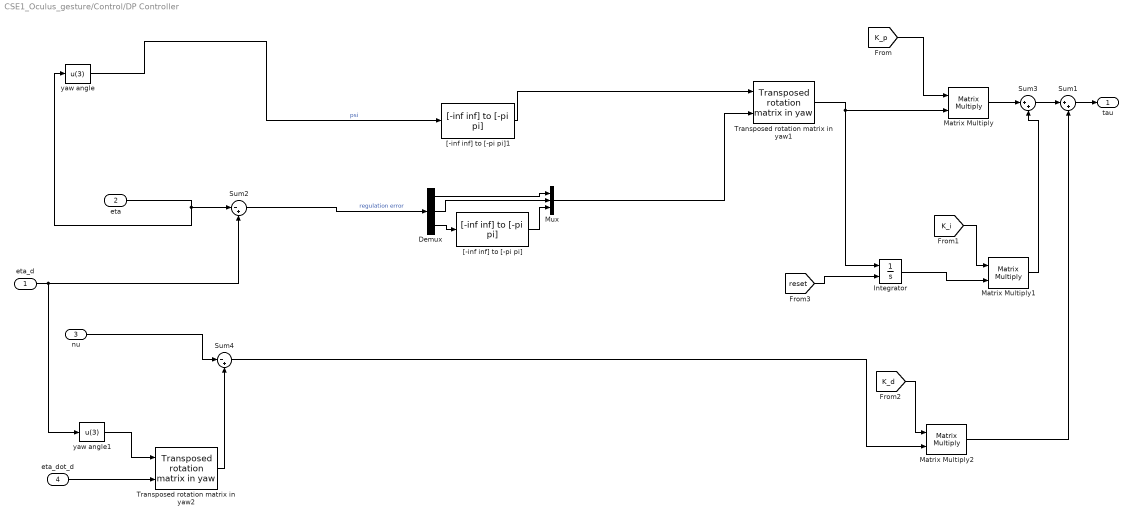
== system CSE1_Oculus_gesture/Control/DP Controller ==
  eta_d : Inport
  eta : Inport  Port=2
  nu : Inport  Port=3
  eta_dot_d : Inport  Port=4
  Demux : Demux  Outputs=3
  Integrator : Integrator  ExternalReset=either
  Matrix Multiply : Product  Multiplication=Matrix(*)
  Matrix Multiply1 : Product  Multiplication=Matrix(*)
  Matrix Multiply2 : Product  Multiplication=Matrix(*)
  Mux : Mux  Inputs=3
  Sum1 : Sum  Inputs=|++  SaturateOnIntegerOverflow=on  InputSameDT=on  OutDataTypeStr=Inherit: Same as first input
  Sum2 : Sum  Inputs=|-+  SaturateOnIntegerOverflow=on  InputSameDT=on  OutDataTypeStr=Inherit: Same as first input
  Sum3 : Sum  Inputs=|++  SaturateOnIntegerOverflow=on  InputSameDT=on  OutDataTypeStr=Inherit: Same as first input
  Sum4 : Sum  Inputs=|-+  SaturateOnIntegerOverflow=on  InputSameDT=on  OutDataTypeStr=Inherit: Same as first input
  Transposed rotation matrix in yaw1 : marine_gnc/Models/ Kinematics/Transposed rotation  matrix in yaw
  Transposed rotation matrix in yaw2 : marine_gnc/Models/ Kinematics/Transposed rotation  matrix in yaw
  "[-inf inf] to [-pi pi]" : marine_gnc/Utilities/Math Operations/[-inf inf] to [-pi pi]
  "[-inf inf] to [-pi pi]1" : marine_gnc/Utilities/Math Operations/[-inf inf] to [-pi pi]
  yaw angle : Fcn  Expr=u(3)
  yaw angle1 : Fcn  Expr=u(3)
  tau : Outport  InitialOutput=0
  wires:
  "[-inf inf] to [-pi pi]1"/1 -> Transposed rotation matrix in yaw1/1
  yaw angle/1 -> "[-inf inf] to [-pi pi]1"/1  "psi"
  Mux/1 -> Transposed rotation matrix in yaw1/2
  Demux/1 -> Mux/1
  Demux/2 -> Mux/2
  "[-inf inf] to [-pi pi]"/1 -> Mux/3
  Sum2/1 -> Demux/1  "regulation error"
  Demux/3 -> "[-inf inf] to [-pi pi]"/1
  Sum1/1 -> tau/1
  eta/1 -> yaw angle/1, Sum2/1
  nu/1 -> Sum4/1
  Matrix Multiply2/1 -> Sum1/2
  Integrator/1 -> Matrix Multiply1/2
  Matrix Multiply/1 -> Sum3/1
  Sum3/1 -> Sum1/1
  Matrix Multiply1/1 -> Sum3/2
  Transposed rotation matrix in yaw1/1 -> Matrix Multiply/2, Integrator/1
  eta_d/1 -> yaw angle1/1, Sum2/2
  [reset] -> Integrator/2
  [K_p] -> Matrix Multiply/1
  [K_i] -> Matrix Multiply1/1
  [K_d] -> Matrix Multiply2/1
  eta_dot_d/1 -> Transposed rotation matrix in yaw2/2
  Transposed rotation matrix in yaw2/1 -> Sum4/2
  Sum4/1 -> Matrix Multiply2/2
  yaw angle1/1 -> Transposed rotation matrix in yaw2/1

== system CSE1_Oculus_gesture/Guidance/Inf,inf tto pi,pi ==
  In1 : Inport
  Demux1 : Demux  Outputs=3
  Mux2 : Mux  Inputs=3
  "[-inf inf] to [-pi pi]" : marine_gnc/Utilities/Math Operations/[-inf inf] to [-pi pi]
  Out1 : Outport
  wires:
  Demux1/1 -> Mux2/1
  Demux1/2 -> Mux2/2
  "[-inf inf] to [-pi pi]"/1 -> Mux2/3
  Demux1/3 -> "[-inf inf] to [-pi pi]"/1
  In1/1 -> Demux1/1
  Mux2/1 -> Out1/1

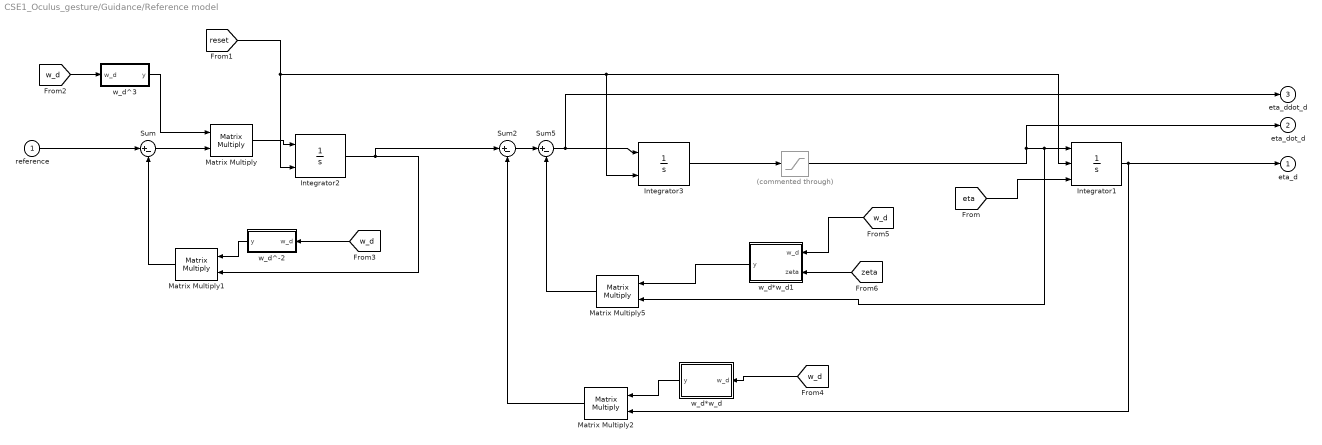
== system CSE1_Oculus_gesture/Guidance/Reference model ==
  reference : Inport
  "       " : Saturate  Commented=through  UpperLimit=[0.3 0.1 1]  LowerLimit=-[0.3 0.1 1]
  Integrator1 : Integrator  ExternalReset=either  InitialConditionSource=external
  Integrator2 : Integrator  ExternalReset=either
  Integrator3 : Integrator  ExternalReset=either
  Matrix Multiply{,1..2,5} (4 alike) : Product  Multiplication=Matrix(*)
  Sum : Sum  Inputs=|+-
  Sum2 : Sum  Inputs=|+-  SaturateOnIntegerOverflow=on  InputSameDT=on  OutDataTypeStr=Inherit: Same as first input
  Sum5 : Sum  Inputs=|+-  SaturateOnIntegerOverflow=on  InputSameDT=on  OutDataTypeStr=Inherit: Same as first input
  w_d*w_d : MATLAB Function  TreatAsAtomicUnit=on
  w_d*w_d1 : MATLAB Function  TreatAsAtomicUnit=on
  w_d^-2 : MATLAB Function  TreatAsAtomicUnit=on
  w_d^3 : MATLAB Function  TreatAsAtomicUnit=on
  eta_d : Outport  InitialOutput=0
  eta_dot_d : Outport  Port=2  InitialOutput=0
  eta_ddot_d : Outport  Port=3  InitialOutput=0
  wires:
  "       "/1 -> Integrator1/1, Matrix Multiply5/2, eta_dot_d/1
  Sum5/1 -> Integrator3/1, eta_ddot_d/1
  Integrator2/1 -> Sum2/1, Matrix Multiply1/2
  Sum2/1 -> Sum5/1
  Matrix Multiply2/1 -> Sum2/2
  Integrator1/1 -> eta_d/1, Matrix Multiply2/2
  Integrator3/1 -> "       "/1
  Matrix Multiply5/1 -> Sum5/2
  reference/1 -> Sum/1
  Sum/1 -> Matrix Multiply/2
  Matrix Multiply/1 -> Integrator2/1
  Matrix Multiply1/1 -> Sum/2
  [w_d] -> w_d^3/1(w_d)
  [w_d] -> w_d^-2/1(w_d)
  [w_d] -> w_d*w_d/1(w_d)
  w_d*w_d/1(y) -> Matrix Multiply2/1
  [zeta] -> w_d*w_d1/2(zeta)
  [w_d] -> w_d*w_d1/1(w_d)
  w_d*w_d1/1(y) -> Matrix Multiply5/1
  [eta] -> Integrator1/3
  [reset] -> Integrator3/2, Integrator1/2, Integrator2/2
  w_d^-2/1(y) -> Matrix Multiply1/1
  w_d^3/1(y) -> Matrix Multiply/1

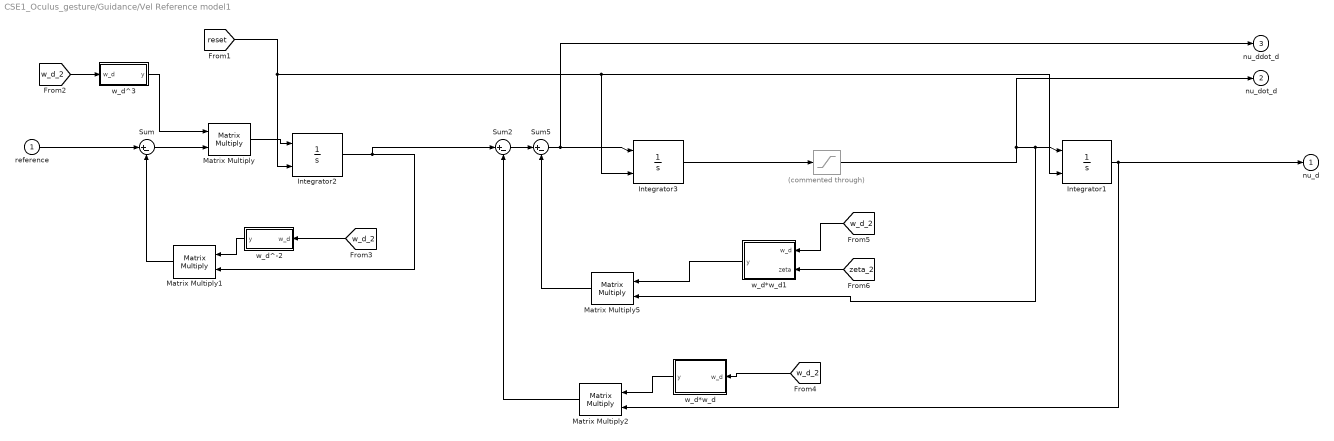
== system CSE1_Oculus_gesture/Guidance/Vel Reference model1 ==
  reference : Inport
  "       " : Saturate  Commented=through  UpperLimit=v_max  LowerLimit=-v_max
  Integrator1 : Integrator  ExternalReset=either
  Integrator2 : Integrator  ExternalReset=either
  Integrator3 : Integrator  ExternalReset=either
  Matrix Multiply{,1..2,5} (4 alike) : Product  Multiplication=Matrix(*)
  Sum : Sum  Inputs=|+-
  Sum2 : Sum  Inputs=|+-  SaturateOnIntegerOverflow=on  InputSameDT=on  OutDataTypeStr=Inherit: Same as first input
  Sum5 : Sum  Inputs=|+-  SaturateOnIntegerOverflow=on  InputSameDT=on  OutDataTypeStr=Inherit: Same as first input
  w_d*w_d : MATLAB Function  TreatAsAtomicUnit=on
  w_d*w_d1 : MATLAB Function  TreatAsAtomicUnit=on
  w_d^-2 : MATLAB Function  TreatAsAtomicUnit=on
  w_d^3 : MATLAB Function  TreatAsAtomicUnit=on
  nu_d : Outport  InitialOutput=0
  nu_dot_d : Outport  Port=2  InitialOutput=0
  nu_ddot_d : Outport  Port=3  InitialOutput=0
  wires:
  "       "/1 -> Integrator1/1, Matrix Multiply5/2, nu_dot_d/1
  Sum5/1 -> Integrator3/1, nu_ddot_d/1
  Integrator2/1 -> Sum2/1, Matrix Multiply1/2
  Sum2/1 -> Sum5/1
  Matrix Multiply2/1 -> Sum2/2
  Integrator1/1 -> Matrix Multiply2/2, nu_d/1
  Integrator3/1 -> "       "/1
  Matrix Multiply5/1 -> Sum5/2
  reference/1 -> Sum/1
  Sum/1 -> Matrix Multiply/2
  Matrix Multiply/1 -> Integrator2/1
  Matrix Multiply1/1 -> Sum/2
  [w_d_2] -> w_d^3/1(w_d)
  [w_d_2] -> w_d^-2/1(w_d)
  [w_d_2] -> w_d*w_d/1(w_d)
  w_d*w_d/1(y) -> Matrix Multiply2/1
  [zeta_2] -> w_d*w_d1/2(zeta)
  [w_d_2] -> w_d*w_d1/1(w_d)
  w_d*w_d1/1(y) -> Matrix Multiply5/1
  [reset] -> Integrator3/2, Integrator1/2, Integrator2/2
  w_d^-2/1(y) -> Matrix Multiply1/1
  w_d^3/1(y) -> Matrix Multiply/1
